simulink model "CCS_Demo"  (R2023b)
settings: Solver=VariableStepAuto  StartTime=0.0  StopTime=Inf  RelTol=1e-3
model workspace (MAT data in the model file):
  SL_ROS_VariableLengthArrays_MaxSizes.CommonInfo.ArrayTruncateAction = 'EmitWarning'
  SL_ROS_VariableLengthArrays_MaxSizes.MsgTypeMap = containers.Map
  SL_ROS_VariableLengthArrays_MaxSizes.MsgTypeMap.serialization.keys = {'sensor_msgs/PointCloud2', 'sensor_msgs/PointField'}
  SL_ROS_VariableLengthArrays_MaxSizes.MsgTypeMap.serialization.values{1}(1).PropertyName = 'Data'
  SL_ROS_VariableLengthArrays_MaxSizes.MsgTypeMap.serialization.values{1}(1).DataType = 'uint8'
  SL_ROS_VariableLengthArrays_MaxSizes.MsgTypeMap.serialization.values{1}(1).MaxLength = 99999999
  SL_ROS_VariableLengthArrays_MaxSizes.MsgTypeMap.serialization.values{1}(2).PropertyName = 'Fields'
  SL_ROS_VariableLengthArrays_MaxSizes.MsgTypeMap.serialization.values{1}(2).DataType = 'sensor_msgs/PointField'
  SL_ROS_VariableLengthArrays_MaxSizes.MsgTypeMap.serialization.values{1}(2).MaxLength = 16
  SL_ROS_VariableLengthArrays_MaxSizes.MsgTypeMap.serialization.values{2}.PropertyName = 'Name'
  SL_ROS_VariableLengthArrays_MaxSizes.MsgTypeMap.serialization.values{2}.DataType = 'uint8'
  SL_ROS_VariableLengthArrays_MaxSizes.MsgTypeMap.serialization.values{2}.MaxLength = 1000000
  SL_ROS_VariableLengthArrays_MaxSizes.MsgTypeMap.serialization.uniformity = 0
  SL_ROS_VariableLengthArrays_MaxSizes.MsgTypeMap.serialization.keyType = 'char'
  SL_ROS_VariableLengthArrays_MaxSizes.MsgTypeMap.serialization.valueType = 'any'
libraries: robotlib x6
settings Model: Creator=lajos  LastModifiedBy=Kuehn

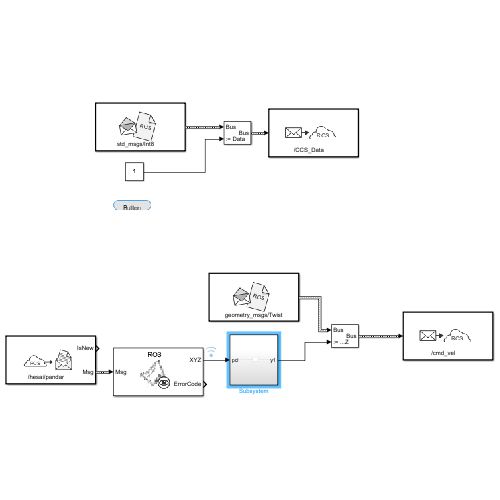
[thumbnail: Simulink's stored preview of the top-level diagram]
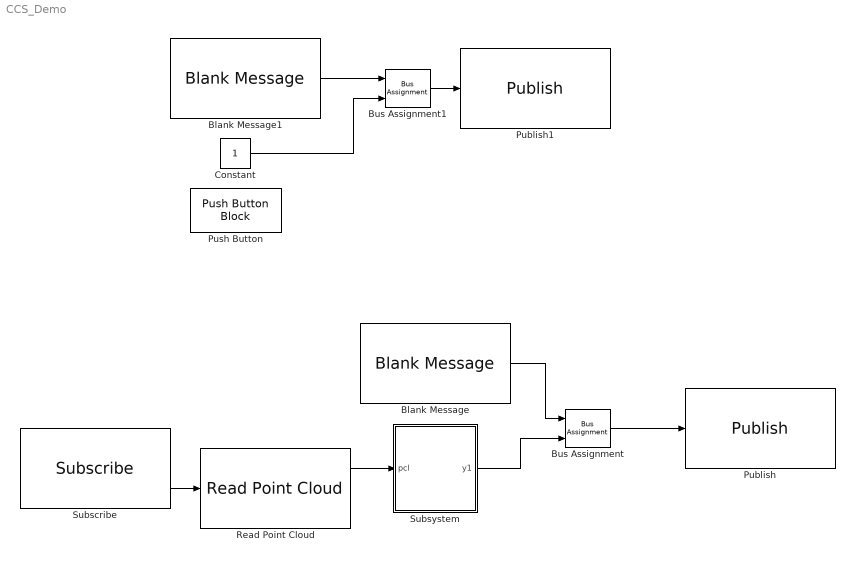
== system CCS_Demo ==
  Blank Message : robotlib/Blank Message  messageClass=Message  entityType=geometry_msgs/Twist  messageType=geometry_msgs/Twist  SampleTime=inf  legacyBusStruct=off
  Blank Message1 : robotlib/Blank Message  messageClass=Message  entityType=std_msgs/Int8  messageType=std_msgs/Int8  SampleTime=inf  legacyBusStruct=off
  Bus Assignment : BusAssignment  AssignedSignals=Angular.Z
  Bus Assignment1 : BusAssignment  AssignedSignals=Data
  Constant : Constant  OutDataTypeStr=int8
  Publish : robotlib/Publish  topicSource=Select from ROS network  topic=/cmd_vel  messageType=geometry_msgs/Twist  legacyBusStruct=off  messageQueueLength=1
  Publish1 : robotlib/Publish  topicSource=Specify your own  topic=/CCS_Data  messageType=std_msgs/Int8  legacyBusStruct=off  messageQueueLength=1
  Push Button : PushButtonBlock  ButtonType=Latch  OffValue=0.000000
  Read Point Cloud : robotlib/Read Point Cloud  MaximumPointCloudSize=[1, 999999]  PreserveStructure=off  ShowRGBOutput=off  ShowIntensityOutput=off  ShowErrorCodeOutput=on  VariableSizeOutputs=off
  Subscribe : robotlib/Subscribe  topicSource=Select from ROS network  topic=/hesai/pandar  messageType=sensor_msgs/PointCloud2  SampleTime=-1  legacyBusStruct=off  messageQueueLength=1
  Subsystem : Subsystem
  wires:
  Subscribe/2 -> Read Point Cloud/1
  Blank Message/1 -> Bus Assignment/1
  Bus Assignment/1 -> Publish/1
  Read Point Cloud/1 -> Subsystem/1(pcl)
  Subsystem/1(y1) -> Bus Assignment/2
  Blank Message1/1 -> Bus Assignment1/1
  Constant/1 -> Bus Assignment1/2
  Bus Assignment1/1 -> Publish1/1

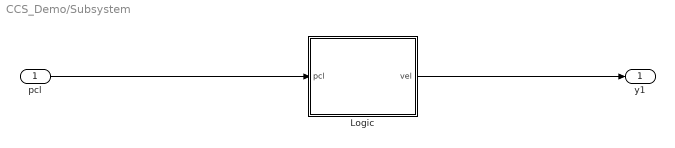
== system CCS_Demo/Subsystem ==
  pcl : Inport
  Logic : MATLAB Function  TreatAsAtomicUnit=on
  y1 : Outport
  wires:
  pcl/1 -> Logic/1(pcl)
  Logic/1(vel) -> y1/1

== matlab function CCS_Demo/Subsystem/Logic ==
  data: pcl input; vel output [0..10]
function vel   = fcn(pcl)


pcl_x = pcl(:, 1);
pcl_y = pcl(:, 2);
pcl_z = pcl(:, 3);

test = pcl(15000, 1);

vel = 0.5;
